simulink model "model2"  (R2020a)
settings: Solver=VariableStepAuto  StartTime=0.0  StopTime=10.0  RelTol=1e-3
settings Model: Creator=hp  LastModifiedBy=hp

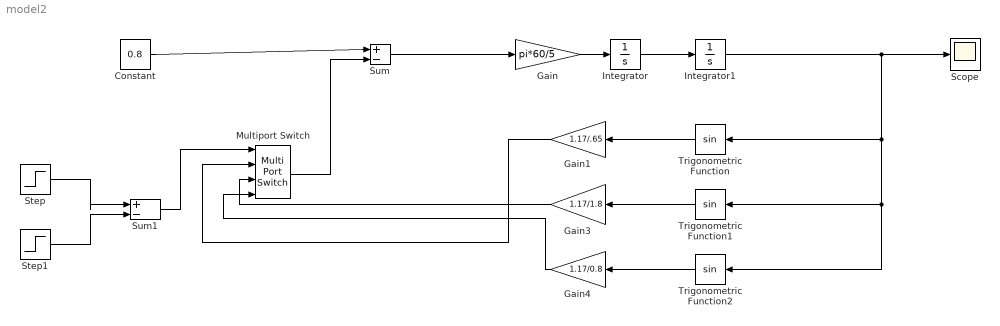
== system model2 ==
  Constant : Constant  Value=0.8
  Gain : Gain  Gain=pi*60/5
  Gain1 : Gain  Gain=1.17/.65
  Gain3 : Gain  Gain=1.17/1.8
  Gain4 : Gain  Gain=1.17/0.8
  Integrator : Integrator
  Integrator1 : Integrator  InitialCondition=26.38*pi/180
  Multiport Switch : MultiPortSwitch
  Scope : Scope
  Step : Step  SampleTime=0
  Step1 : Step  Time=1.26  SampleTime=0
  Sum : Sum  Inputs=|+-
  Sum1 : Sum  Inputs=|+-
  Trigonometric Function : Trigonometry
  Trigonometric Function1 : Trigonometry
  Trigonometric Function2 : Trigonometry
  wires:
  Multiport Switch/1 -> Sum/2
  Step1/1 -> Sum1/2
  Step/1 -> Sum1/1
  Sum1/1 -> Multiport Switch/1
  Trigonometric Function/1 -> Gain1/1
  Sum/1 -> Gain/1
  Constant/1 -> Sum/1
  Gain/1 -> Integrator/1
  Integrator/1 -> Integrator1/1
  Integrator1/1 -> Trigonometric Function2/1, Trigonometric Function1/1, Trigonometric Function/1, Scope/1
  Trigonometric Function1/1 -> Gain3/1
  Gain1/1 -> Multiport Switch/2
  Gain3/1 -> Multiport Switch/3
  Gain4/1 -> Multiport Switch/4
  Trigonometric Function2/1 -> Gain4/1
